simulink model "CostasLoop"  (R2020a)
settings: Solver=ode45  StartTime=0.0  StopTime=5000  RelTol=1e-3  EnableMultiTasking=on
PreLoadFcn:
  | CostasLoop_PreLoadFcn
values from neighbouring files (symbols this model uses):
  h = hh    [CostasLoop_PreLoadFcn.m]
  k_i = (4*theta_0*theta_0)/(1+2*eta*theta_0+theta_0*theta_0)    [CostasLoop_PreLoadFcn.m]
  k_p = (4*eta*theta_0)/(1+2*eta*theta_0+theta_0*theta_0)    [CostasLoop_PreLoadFcn.m]
libraries: xbsIndex_r4 x34, dspmlti4 x2, xbsCopyrightNotice_r4 x1, simulink x1
settings Model: ExtModeTrigMode=oneshot  ExtModeArmWhenConnect=off  Creator=alexc  LastModifiedBy=viswanad
settings DataIOCC: SaveFormat=Array  SignalLoggingSaveFormat=ModelDataLogs  ReturnWorkspaceOutputs=off  SignalLoggingName=sigsOut
settings OptimizationCC: BlockReduction=off  BooleanDataType=off  DefaultParameterBehavior=Inlined  ExpressionDepthLimit=2147483647  InitFltsAndDblsToZero=on  LifeSpan=inf
settings DebuggingCC: SaveWithParameterizedLinksMsg=none  UnderspecifiedInitializationDetection=Classic  MergeDetectMultiDrivingBlocksExec=none  SignalResolutionControl=TryResolveAllWithWarning  MultiTaskDSMMsg=warning  MultiTaskCondExecSysMsg=none  FcnCallInpInsideContextMsg=warning  StateNameClashWarn=warning  SFUnexpectedBacktrackingDiag=warning  SFNoUnconditionalDefaultTransitionDiag=warning  SFExecutionAtInitializationDiag=none  ArithmeticOperatorsInVariantConditions=warning
settings HardwareCC: ProdBitPerPointer=32  ProdBitPerSizeT=32  ProdBitPerPtrDiffT=32  ProdLargestAtomicFloat=None  ProdIntDivRoundTo=Undefined  ProdEndianess=Unspecified  ProdWordSize=32  ProdHWDeviceType=32-bit Generic  TargetUnknown=on
settings ModelReferenceCC: PropagateSignalLabelsOutOfModel=off
settings SFSimCC: SimUseLocalCustomCode=off  CustomCodeUndefinedFunction=UseInterfaceOnly
settings RTWCC: Description=Generic Real-Time Target  RTWUseLocalCustomCode=off
settings CodeAppCC: StateflowObjectComments=on
settings GRTTargetCC: TargetFcnLib=ansi_tfl_tmw.mat  TargetLangStandard=C89/C90 (ANSI)  CombineOutputUpdateFcns=off  GRTInterface=on
settings ConfigComp: CovMetricSettings=dw  CovSaveCumulativeToWorkspaceVar=on  CovSaveSingleToWorkspaceVar=on  CovExternalEMLEnable=off

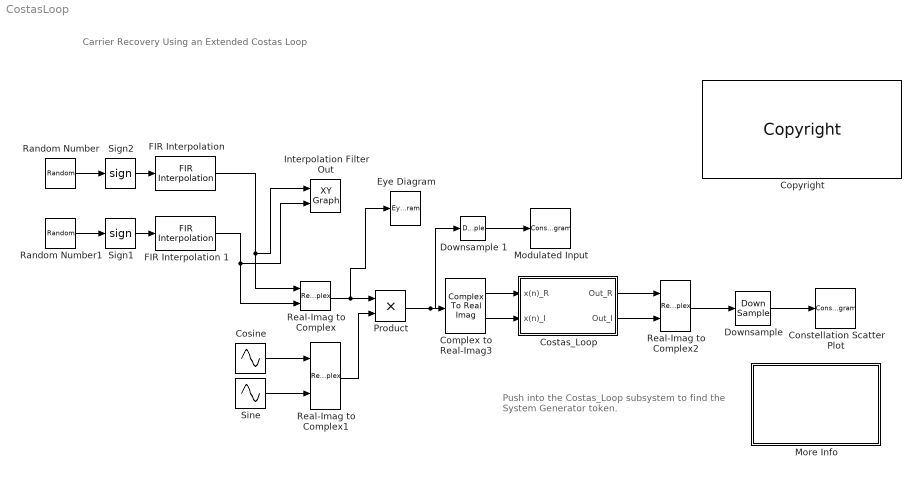
== system CostasLoop ==
  note: Carrier Recovery Using an Extended Costas Loop
  note: Push into the Costas_Loop subsystem
      | to find the System Generator token.
  " Eye Diagram" : EyeDiagram  Tag=EyeDiagram
  Complex to Real-Imag3 : ComplexToRealImag
  Constellation Scatter Plot : ConstellationDiagram  Tag=ScatterPlot
  Copyright : xbsCopyrightNotice_r4/Copyright  copyrighttext="Copyright (c) 2021  by  Xilinx, Inc. All rights reserved.<br><br>This file contains proprietary, confidential information of Xilinx, Inc., is distributed under license from Xilinx, Inc., and may be used, copied and/or disclosed only pursuant to the terms of a valid license agreement with Xilinx, Inc. Xilinx hereby grants you a license to use this file solely for design, simulation, implementation and creation of design files limited to Xilinx devices or technologies. Use with non-Xilinx devices or technologies is expressly prohibited and immediately terminates your license unless covered by a separate agreement.<br><br>Xilinx is providing this design, code, or information \"as-is\" solely for use in developing programs and solutions for Xilinx devices, with no obligation on the part of Xilinx to provide support. By providing this design, code, or information as one possible implementation of this feature, application or standard, Xilinx is making no representation that this implementation is free from any claims of infringement. You are responsible for obtaining any rights you may require for your implementation. Xilinx expressly disclaims any warranty whatsoever with respect to the adequacy of the implementation, including but not limited to any warranties or representations that this implementation is free from claims of infringement, implied warranties of merchantability or fitness for a particular purpose.<br><br>Xilinx products are not intended for use in life support appliances, devices, or systems. Use in such applications is expressly prohibited.<br><br>Any modifications that are made to the Source Code are done at the user's sole risk and will be unsupported.<br><br>This copyright and support notice must be retained as part of this text at all times. (c) Copyright 1995-2021 Xilinx, Inc. All rights reserved."  block_type=copyright
  Cosine : Sin  Frequency=2*pi*0.001/8  Phase=pi/2  SampleTime=8
  Costas_Loop : Subsystem
  "Downsample " : DownSample  N=8  InputProcessing=Inherited (this choice will be removed - see release notes)  RateOptions=Allow multirate processing
  Downsample 1 : DownSample  N=8  phase=2  InputProcessing=Inherited (this choice will be removed - see release notes)  RateOptions=Allow multirate processing
  "FIR Interpolation " : dspmlti4/FIR Interpolation  FilterSource=Dialog parameters  PrivateCoeffs=0  h=[h]  L=8  FilterObject=Hm_firinterp  InputProcessing=Columns as channels (frame based)  framing=Allow multirate processing  outputBufInitCond=0  roundingMode=Floor  overflowMode=off  firstCoeffDataTypeStr=Inherit: Same word length as input  firstCoeffMin=[]  firstCoeffMax=[]  firstCoeffLastDataTypeStr=Inherit: Same word length as input  outputDataTypeStr=Inherit: Same as accumulator  outputMin=[]  outputMax=[]  outputLastDataTypeStr=Inherit: Same as accumulator
  FIR Interpolation 1 : dspmlti4/FIR Interpolation  FilterSource=Dialog parameters  PrivateCoeffs=0  h=[h]  L=8  FilterObject=Hm_firinterp  InputProcessing=Columns as channels (frame based)  framing=Allow multirate processing  outputBufInitCond=0  roundingMode=Floor  overflowMode=off  firstCoeffDataTypeStr=Inherit: Same word length as input  firstCoeffMin=[]  firstCoeffMax=[]  firstCoeffLastDataTypeStr=Inherit: Same word length as input  outputDataTypeStr=Inherit: Same as accumulator  outputMin=[]  outputMax=[]  outputLastDataTypeStr=Inherit: Same as accumulator
  Interpolation Filter Out : simulink/Sinks/XY Graph  xmin=-1.75  xmax=1.75  ymin=-1.75  ymax=1.75  st=-1
  Modulated Input : ConstellationDiagram  Tag=ScatterPlot
  More Info : Subsystem
      mask Display: disp('Double click\n for\n more information.')
  Product : Product  InputSameDT=on  SaturateOnIntegerOverflow=on  OutDataTypeStr=Inherit: Same as first input
  Random Number : RandomNumber  SampleTime=8
  Random Number1 : RandomNumber  Seed=2  SampleTime=8
  Real-Imag to Complex : RealImagToComplex
  Real-Imag to Complex1 : RealImagToComplex
  Real-Imag to Complex2 : RealImagToComplex
  Sign1 : Signum
  Sign2 : Signum
  Sine : Sin  Frequency=2*pi*0.001/8  SampleTime=8
  wires:
  Sign1/1 -> FIR Interpolation 1/1
  Sign2/1 -> "FIR Interpolation "/1
  Real-Imag to Complex/1 -> Product/1, " Eye Diagram"/1
  Product/1 -> Complex to Real-Imag3/1, Downsample 1/1
  Costas_Loop/1(Out_R) -> Real-Imag to Complex2/1
  Costas_Loop/2(Out_I) -> Real-Imag to Complex2/2
  Real-Imag to Complex1/1 -> Product/2
  Cosine/1 -> Real-Imag to Complex1/1
  Downsample 1/1 -> Modulated Input/1
  Random Number/1 -> Sign2/1
  Random Number1/1 -> Sign1/1
  Complex to Real-Imag3/1 -> Costas_Loop/1(x(n)_R)
  Complex to Real-Imag3/2 -> Costas_Loop/2(x(n)_I)
  Real-Imag to Complex2/1 -> "Downsample "/1
  Sine/1 -> Real-Imag to Complex1/2
  "FIR Interpolation "/1 -> Real-Imag to Complex/1, Interpolation Filter Out/1
  FIR Interpolation 1/1 -> Real-Imag to Complex/2, Interpolation Filter Out/2
  "Downsample "/1 -> Constellation Scatter Plot/1

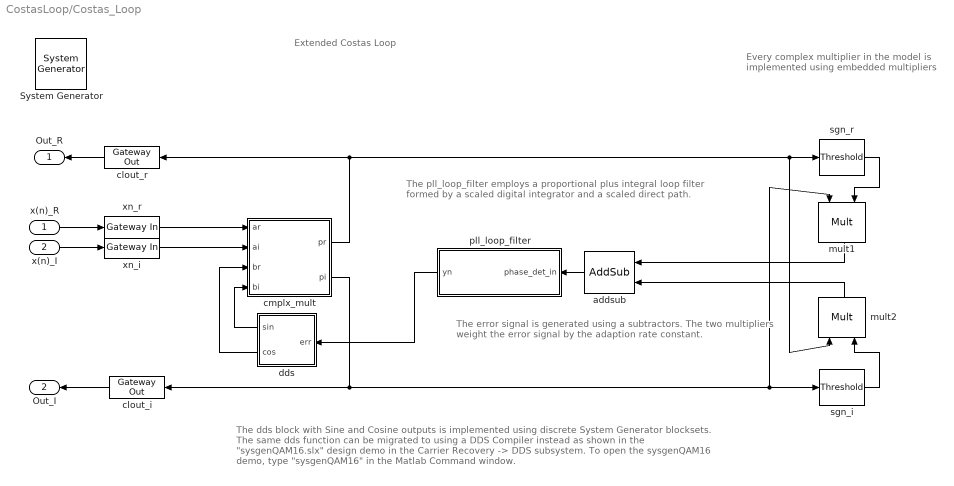
== system CostasLoop/Costas_Loop ==
  note: Extended Costas Loop
  note: The error signal is generated using a subtractors.  The
      | two multipliers weight  the error signal by the adaption
      | rate constant.
  note: The pll_loop_filter employs a proportional plus integral
      | loop filter formed by a scaled digital integrator
      | and a scaled direct path.
  note: Every complex multiplier in the model is
      | implemented using embedded multipliers
  note: The dds block with Sine and Cosine outputs is implemented using discrete System Generator blocksets.
      | The same dds function can be migrated to using a DDS Compiler instead as shown in the "sysgenQAM16.slx"
      | design demo in the Carrier Recovery -> DDS subsystem. To open the sysgenQAM16 demo, type "sysgenQAM16"
      | in the Matlab Command window.
  x(n)_R : Inport
  x(n)_I : Inport  Port=2
  " System Generator" : xbsIndex_r4/ System Generator  Tag=genX  xilinxfamily=kintex7  part=xc7k325t  speed=-3  package=fbg676  synthesis_tool=Vivado  clock_wrapper=Clock Enables  directory=./netlist  proj_type=Project Navigator  Synth_file=XST Defaults  Impl_file=ISE Defaults  testbench=off  simulink_period=1  sysclk_period=25  dcm_input_clock_period=100  incr_netlist=off  trim_vbits=Everywhere in SubSystem  dbl_ovrd=According to Block Masks  core_generation=According to Block Masks  run_coregen=off  deprecated_control=off  eval_field=0  block_type=sysgen
      settings: block_version=9.2-dev
  addsub : xbsIndex_r4/AddSub  mode=Subtraction  use_carryin=off  use_carryout=off  en=off  latency=0  precision=User Defined  arith_type="Signed  (2's comp)"  n_bits=16  bin_pt=13  quantization="Round  (unbiased: +/- Inf)"  overflow=Saturate  use_behavioral_HDL=on  hw_selection=Fabric  pipelined=off  use_rpm=off  XmcBlockStatus=1  maskContainerNames=tabcontainer1  block_type=addsub  block_config=sysgen:Addsub_config
  clout_i : xbsIndex_r4/Gateway Out  inherit_from_input=off  hdl_port=on  rows=1  columns=1  UseAsDAC=off  DACChannel='1'  interface=None  automatic_assignment=on  address_offset=hex2dec('00')  intf_name=''  intf_description=''  timing_constraint=None  locs_specified=off  LOCs={}  io_standard={}  XmcBlockStatus=1  maskContainerNames=group4  block_type=gatewayout  block_config=sysgen:gateway_out_config
  clout_r : xbsIndex_r4/Gateway Out  inherit_from_input=off  hdl_port=on  rows=1  columns=1  UseAsDAC=off  DACChannel='1'  interface=None  automatic_assignment=on  address_offset=hex2dec('00')  intf_name=''  intf_description=''  timing_constraint=None  locs_specified=off  LOCs={}  io_standard={}  XmcBlockStatus=1  maskContainerNames=group4  block_type=gatewayout  block_config=sysgen:gateway_out_config
  cmplx_mult : Subsystem
  dds : Subsystem
  mult1 : xbsIndex_r4/Mult  precision=User Defined  arith_type="Signed  (2's comp)"  n_bits=16  bin_pt=13  quantization="Round  (unbiased: +/- Inf)"  overflow=Wrap  en=off  latency=0  use_behavioral_HDL=off  opt=Speed  use_embedded=on  optimum_pipeline=off  pipeline=off  use_rpm=off  placement_style=Rectangular shape  XmcBlockStatus=1  maskContainerNames=group1  block_type=mult  block_config=sysgen:Mult_config
  mult2 : xbsIndex_r4/Mult  precision=User Defined  arith_type="Signed  (2's comp)"  n_bits=16  bin_pt=13  quantization="Round  (unbiased: +/- Inf)"  overflow=Wrap  en=off  latency=0  use_behavioral_HDL=off  opt=Speed  use_embedded=on  optimum_pipeline=off  pipeline=off  use_rpm=off  placement_style=Rectangular shape  XmcBlockStatus=1  maskContainerNames=group1  block_type=mult  block_config=sysgen:Mult_config
  pll_loop_filter : Subsystem
  sgn_i : xbsIndex_r4/Threshold  en=off  latency=0  XmcBlockStatus=1  maskContainerNames=group2  block_type=sgn  block_config=sysgen:Sgn_config
  sgn_r : xbsIndex_r4/Threshold  en=off  latency=0  XmcBlockStatus=1  maskContainerNames=group2  block_type=sgn  block_config=sysgen:Sgn_config
  xn_i : xbsIndex_r4/Gateway In  gui_display_data_type=Fixed-point  arith_type=Signed (2's comp)  n_bits=8  bin_pt=6  preci_type=Single  exp_width=8  frac_width=24  rows=1  columns=1  quantization="Round  (unbiased: +/- Inf)"  overflow=Saturate  period=1  UseAsADC=off  ADCChannel='1'  interface=None  automatic_assignment=on  address_offset=hex2dec('00')  intf_name=''  intf_description=''  default_value=0  timing_constraint=None  locs_specified=off  LOCs={}  io_standard={}  inherit_from_input=off  hdl_port=on  XmcBlockStatus=1  maskContainerNames=group4  block_type=gatewayin  block_config=sysgen:gateway_in_config
  xn_r : xbsIndex_r4/Gateway In  gui_display_data_type=Fixed-point  arith_type=Signed (2's comp)  n_bits=8  bin_pt=6  preci_type=Single  exp_width=8  frac_width=24  rows=1  columns=1  quantization="Round  (unbiased: +/- Inf)"  overflow=Saturate  period=1  UseAsADC=off  ADCChannel='1'  interface=None  automatic_assignment=on  address_offset=hex2dec('00')  intf_name=''  intf_description=''  default_value=0  timing_constraint=None  locs_specified=off  LOCs={}  io_standard={}  inherit_from_input=off  hdl_port=on  XmcBlockStatus=1  maskContainerNames=group4  block_type=gatewayin  block_config=sysgen:gateway_in_config
  Out_R : Outport
  Out_I : Outport  Port=2
  wires:
  clout_r/1 -> Out_R/1
  cmplx_mult/1(pr) -> mult2/1, sgn_r/1, clout_r/1
  mult2/1 -> addsub/2
  mult1/1 -> addsub/1
  addsub/1 -> pll_loop_filter/1(phase_det_in)
  sgn_r/1 -> mult1/2
  sgn_i/1 -> mult2/2
  dds/1(sin) -> cmplx_mult/4(bi)
  pll_loop_filter/1(yn) -> dds/1(err)
  clout_i/1 -> Out_I/1
  cmplx_mult/2(pi) -> clout_i/1, mult1/1, sgn_i/1
  dds/2(cos) -> cmplx_mult/3(br)
  x(n)_I/1 -> xn_i/1
  xn_i/1 -> cmplx_mult/2(ai)
  x(n)_R/1 -> xn_r/1
  xn_r/1 -> cmplx_mult/1(ar)

== system CostasLoop/More Info ==
  note: This design shows an implementation of Costas Loop used for Carrier Recovery.
      | The modulated input is modeled using simulink blocks while the costas loop
      | algorithm is implemented using System Generator for DSP blocks.
      |
      | The dds block with Sine and Cosine outputs is implemented using basic
      | System Generator Blocks.The pll_loop_filter employs a proportional plus integral
      | loop filter formed by a scaled digital integrator and a scaled direct path. The error
      | signal is generated using a subtractors.  Two multipliers weight  the error signal
      | by the adaption rate constant.
      |
      |
      | For additional information on Costas Loop:
      |
      | Simon Haykin,  "Communication Systems", 4th Edition, pp. 453-454.
  note: Carrier Recovery Using an Extended Costas Loop

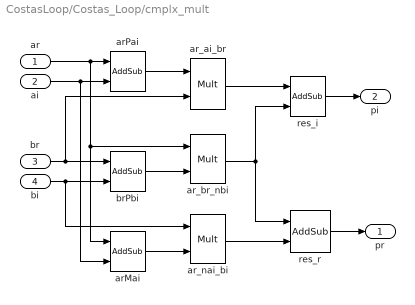
== system CostasLoop/Costas_Loop/cmplx_mult ==
  ar : Inport
  ai : Inport  Port=2
  br : Inport  Port=3
  bi : Inport  Port=4
  arMai : xbsIndex_r4/AddSub  mode=Subtraction  use_carryin=off  use_carryout=off  en=off  latency=0  precision=User Defined  arith_type="Signed  (2's comp)"  n_bits=17  bin_pt=13  quantization="Round  (unbiased: +/- Inf)"  overflow=Saturate  use_behavioral_HDL=on  hw_selection=Fabric  pipelined=off  use_rpm=off  XmcBlockStatus=1  maskContainerNames=tabcontainer1  block_type=addsub  block_config=sysgen:Addsub_config
  arPai : xbsIndex_r4/AddSub  mode=Addition  use_carryin=off  use_carryout=off  en=off  latency=0  precision=Full  arith_type="Signed  (2's comp)"  n_bits=17  bin_pt=13  quantization="Round  (unbiased: +/- Inf)"  overflow=Saturate  use_behavioral_HDL=on  hw_selection=Fabric  pipelined=off  use_rpm=off  XmcBlockStatus=1  maskContainerNames=tabcontainer1  block_type=addsub  block_config=sysgen:Addsub_config
  ar_ai_br : xbsIndex_r4/Mult  precision=User Defined  arith_type="Signed  (2's comp)"  n_bits=16  bin_pt=13  quantization="Round  (unbiased: +/- Inf)"  overflow=Saturate  en=off  latency=0  use_behavioral_HDL=off  opt=Speed  use_embedded=on  optimum_pipeline=off  pipeline=off  use_rpm=off  placement_style=Rectangular shape  XmcBlockStatus=1  maskContainerNames=group1  block_type=mult  block_config=sysgen:Mult_config
  ar_br_nbi : xbsIndex_r4/Mult  precision=User Defined  arith_type="Signed  (2's comp)"  n_bits=16  bin_pt=13  quantization="Round  (unbiased: +/- Inf)"  overflow=Saturate  en=off  latency=0  use_behavioral_HDL=off  opt=Speed  use_embedded=on  optimum_pipeline=off  pipeline=off  use_rpm=off  placement_style=Rectangular shape  XmcBlockStatus=1  maskContainerNames=group1  block_type=mult  block_config=sysgen:Mult_config
  ar_nai_bi : xbsIndex_r4/Mult  precision=User Defined  arith_type="Signed  (2's comp)"  n_bits=16  bin_pt=13  quantization="Round  (unbiased: +/- Inf)"  overflow=Saturate  en=off  latency=0  use_behavioral_HDL=off  opt=Speed  use_embedded=on  optimum_pipeline=off  pipeline=off  use_rpm=off  placement_style=Rectangular shape  XmcBlockStatus=1  maskContainerNames=group1  block_type=mult  block_config=sysgen:Mult_config
  brPbi : xbsIndex_r4/AddSub  mode=Subtraction  use_carryin=off  use_carryout=off  en=off  latency=0  precision=Full  arith_type="Signed  (2's comp)"  n_bits=17  bin_pt=13  quantization="Round  (unbiased: +/- Inf)"  overflow=Saturate  use_behavioral_HDL=on  hw_selection=Fabric  pipelined=off  use_rpm=off  XmcBlockStatus=1  maskContainerNames=tabcontainer1  block_type=addsub  block_config=sysgen:Addsub_config
  res_i : xbsIndex_r4/AddSub  mode=Subtraction  use_carryin=off  use_carryout=off  en=off  latency=0  precision=User Defined  arith_type="Signed  (2's comp)"  n_bits=17  bin_pt=13  quantization="Round  (unbiased: +/- Inf)"  overflow=Saturate  use_behavioral_HDL=on  hw_selection=Fabric  pipelined=off  use_rpm=off  XmcBlockStatus=1  maskContainerNames=tabcontainer1  block_type=addsub  block_config=sysgen:Addsub_config
  res_r : xbsIndex_r4/AddSub  mode=Addition  use_carryin=off  use_carryout=off  en=off  latency=0  precision=User Defined  arith_type="Signed  (2's comp)"  n_bits=17  bin_pt=13  quantization="Round  (unbiased: +/- Inf)"  overflow=Saturate  use_behavioral_HDL=on  hw_selection=Fabric  pipelined=off  use_rpm=off  XmcBlockStatus=1  maskContainerNames=tabcontainer1  block_type=addsub  block_config=sysgen:Addsub_config
  pr : Outport
  pi : Outport  Port=2
  wires:
  res_r/1 -> pr/1
  ar_nai_bi/1 -> res_r/2
  arMai/1 -> ar_nai_bi/2
  res_i/1 -> pi/1
  ar_ai_br/1 -> res_i/1
  ar_br_nbi/1 -> res_r/1, res_i/2
  brPbi/1 -> ar_br_nbi/2
  arPai/1 -> ar_ai_br/1
  bi/1 -> ar_nai_bi/1, brPbi/2
  br/1 -> ar_ai_br/2, brPbi/1
  ai/1 -> arMai/2, arPai/2
  ar/1 -> ar_br_nbi/1, arMai/1, arPai/1

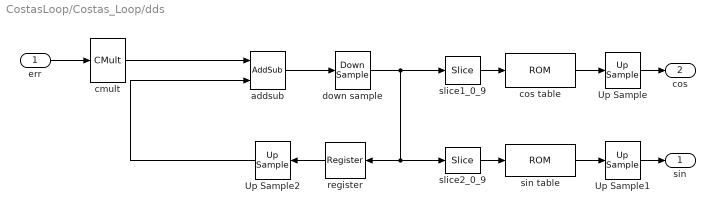
== system CostasLoop/Costas_Loop/dds ==
  err : Inport
  Up Sample : xbsIndex_r4/Up Sample  sample_ratio=64  copy_samples=on  en=off  latency=0  XmcBlockStatus=1  maskContainerNames=group1  block_type=usamp  block_config=sysgen:Upsample_config
  Up Sample1 : xbsIndex_r4/Up Sample  sample_ratio=64  copy_samples=on  en=off  latency=0  XmcBlockStatus=1  maskContainerNames=group1  block_type=usamp  block_config=sysgen:Upsample_config
  Up Sample2 : xbsIndex_r4/Up Sample  sample_ratio=64  copy_samples=on  en=off  latency=0  XmcBlockStatus=1  maskContainerNames=group1  block_type=usamp  block_config=sysgen:Upsample_config
  addsub : xbsIndex_r4/AddSub  mode=Addition  use_carryin=off  use_carryout=off  en=off  latency=0  precision=User Defined  arith_type="Signed  (2's comp)"  n_bits=32  bin_pt=0  quantization="Round  (unbiased: +/- Inf)"  overflow=Wrap  use_behavioral_HDL=on  hw_selection=Fabric  pipelined=off  use_rpm=off  XmcBlockStatus=1  maskContainerNames=tabcontainer1  block_type=addsub  block_config=sysgen:Addsub_config
  cmult : xbsIndex_r4/CMult  const=1024  gui_display_data_type=Fixed-point  const_n_bits=16  const_bin_pt=0  float_type=Single  exp_bits=8  fraction_bits=24  en=off  latency=0  precision=User Defined  arith_type="Signed  (2's comp)"  n_bits=32  bin_pt=0  quantization=Truncate  overflow=Wrap  use_behavioral_HDL=off  mem_type=Distributed RAM  pipeline=off  use_rpm=off  placement_style=Rectangular Shape  XmcBlockStatus=1  maskContainerNames=tabcontainer1  block_type=cmult  block_config=sysgen:CMult_config
      settings: infoedit=[]
  cos table : xbsIndex_r4/ROM  depth=1024  initVector=cos([0:1023]*2*pi/1024)  distributed_mem=Block RAM  rst=off  init_reg=0  en=off  latency=1  optimize_latency=off  gui_display_data_type=Fixed-point  arith_type="Signed  (2's comp)"  n_bits=8  bin_pt=6  preci_type=Single  exp_width=8  frac_width=24  optimize=Area  use_rpm=off  simulation_type=fast_sim  XmcBlockStatus=1  maskContainerNames=tabcontainer1  block_type=sprom  block_config=sysgen:SPROM_config
  down sample : xbsIndex_r4/Down Sample  sample_ratio=64  sample_phase=First Value of Frame  en=off  rst=off  latency=0  XmcBlockStatus=1  maskContainerNames=group1  block_type=dsamp  block_config=sysgen:Downsample_config
  register : xbsIndex_r4/Register  init=0  rst=off  en=off  XmcBlockStatus=1  maskContainerNames=tabcontainer1  block_type=register  block_config=sysgen:Register_config
  sin table : xbsIndex_r4/ROM  depth=1024  initVector=-sin([0:1023]*2*pi/1024)  distributed_mem=Block RAM  rst=off  init_reg=0  en=off  latency=1  optimize_latency=off  gui_display_data_type=Fixed-point  arith_type="Signed  (2's comp)"  n_bits=8  bin_pt=6  preci_type=Single  exp_width=8  frac_width=24  optimize=Area  use_rpm=off  simulation_type=fast_sim  XmcBlockStatus=1  maskContainerNames=tabcontainer1  block_type=sprom  block_config=sysgen:SPROM_config
  slice1_0_9 : xbsIndex_r4/Slice  nbits=10  boolean_output=off  mode=Lower Bit Location + Width  bit1=0  base1=MSB of Input  bit0=0  base0=LSB of Input  XmcBlockStatus=1  maskContainerNames=group1  block_type=slice  block_config=sysgen:Slice_config
  slice2_0_9 : xbsIndex_r4/Slice  nbits=10  boolean_output=off  mode=Lower Bit Location + Width  bit1=0  base1=MSB of Input  bit0=0  base0=LSB of Input  XmcBlockStatus=1  maskContainerNames=group1  block_type=slice  block_config=sysgen:Slice_config
  sin : Outport
  cos : Outport  Port=2
  wires:
  err/1 -> cmult/1
  cmult/1 -> addsub/1
  addsub/1 -> down sample/1
  down sample/1 -> slice1_0_9/1, slice2_0_9/1, register/1
  slice1_0_9/1 -> cos table/1
  slice2_0_9/1 -> sin table/1
  cos table/1 -> Up Sample/1
  Up Sample/1 -> cos/1
  sin table/1 -> Up Sample1/1
  Up Sample1/1 -> sin/1
  Up Sample2/1 -> addsub/2
  register/1 -> Up Sample2/1

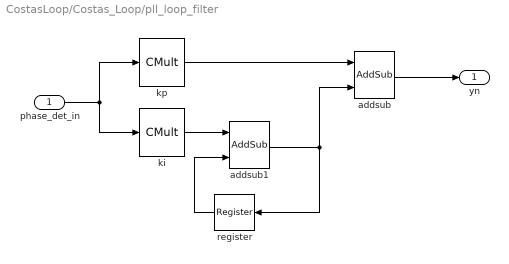
== system CostasLoop/Costas_Loop/pll_loop_filter ==
  phase_det_in : Inport
  addsub : xbsIndex_r4/AddSub  mode=Addition  use_carryin=off  use_carryout=off  en=off  latency=0  precision=User Defined  arith_type=Unsigned  n_bits=32  bin_pt=28  quantization="Round  (unbiased: +/- Inf)"  overflow=Wrap  use_behavioral_HDL=on  hw_selection=Fabric  pipelined=off  use_rpm=off  XmcBlockStatus=1  maskContainerNames=tabcontainer1  block_type=addsub  block_config=sysgen:Addsub_config
  addsub1 : xbsIndex_r4/AddSub  mode=Addition  use_carryin=off  use_carryout=off  en=off  latency=0  precision=User Defined  arith_type="Signed  (2's comp)"  n_bits=32  bin_pt=28  quantization="Round  (unbiased: +/- Inf)"  overflow=Wrap  use_behavioral_HDL=on  hw_selection=Fabric  pipelined=off  use_rpm=off  XmcBlockStatus=1  maskContainerNames=tabcontainer1  block_type=addsub  block_config=sysgen:Addsub_config
  ki : xbsIndex_r4/CMult  const=k_i  gui_display_data_type=Fixed-point  const_n_bits=16  const_bin_pt=15  float_type=Single  exp_bits=8  fraction_bits=24  en=off  latency=0  precision=User Defined  arith_type="Signed  (2's comp)"  n_bits=32  bin_pt=28  quantization="Round  (unbiased: +/- Inf)"  overflow=Wrap  use_behavioral_HDL=off  mem_type=Distributed RAM  pipeline=off  use_rpm=off  placement_style=Rectangular Shape  XmcBlockStatus=1  maskContainerNames=tabcontainer1  block_type=cmult  block_config=sysgen:CMult_config
      settings: infoedit=[]
  kp : xbsIndex_r4/CMult  const=k_p  gui_display_data_type=Fixed-point  const_n_bits=16  const_bin_pt=15  float_type=Single  exp_bits=8  fraction_bits=24  en=off  latency=0  precision=User Defined  arith_type="Signed  (2's comp)"  n_bits=32  bin_pt=28  quantization="Round  (unbiased: +/- Inf)"  overflow=Wrap  use_behavioral_HDL=off  mem_type=Distributed RAM  pipeline=off  use_rpm=off  placement_style=Rectangular Shape  XmcBlockStatus=1  maskContainerNames=tabcontainer1  block_type=cmult  block_config=sysgen:CMult_config
      settings: infoedit=[]
  register : xbsIndex_r4/Register  init=0  rst=off  en=off  XmcBlockStatus=1  maskContainerNames=tabcontainer1  block_type=register  block_config=sysgen:Register_config
  yn : Outport
  wires:
  ki/1 -> addsub1/1
  phase_det_in/1 -> ki/1, kp/1
  register/1 -> addsub1/2
  addsub1/1 -> addsub/2, register/1
  kp/1 -> addsub/1
  addsub/1 -> yn/1
